simulink model "untitled1"  (Simulink 7.9)
settings: Solver=ode45  StartTime=0.0  StopTime=10.0  RelTol=1e-3
undefined symbols (not defined in the file or in its folder): b0, b1, b2, b3, Cyclic, D, dBW, F_nco, Fs, Hz, magnitude, N, nco_nominal, OFDM_Frame, sided, Ts, Two
libraries: dspobslib x17, dspsigops x8, simulink x8, dspsnks4 x4, dspxfrm3 x3, dspsrcs4 x3, dspstat3 x3, dspbuff3 x2, dsppolyfun x1, commrandsrc2 x1, commsink2 x1
settings Model: Creator=Estilo  LastModifiedBy=Estilo

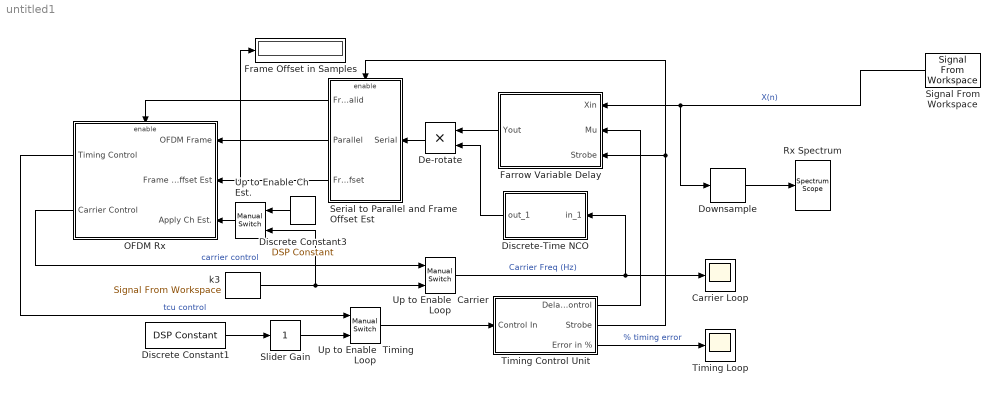
== system untitled1 ==
  Carrier Loop : Scope
      settings: TimeRange=0.008999999999999999  YMin=-1000  YMax=1000  MaxDataPoints=50000  Decimation=4
  De-rotate : Product  RndMeth=Zero
  Discrete Constant1 : dspobslib/DSP Constant  Value=nco_nominal  SampleMode=Discrete  discreteOutput=Sample-based (interpret vectors as 1-D)  continuousOutput=Sample-based  sampTime=2/F_nco  framePeriod=2/F_nco  dataType=Inherit via back propagation  isSigned=on  wordLen=16  udDataType=sfix(16)  fracBitsMode=Best precision  numFracBits=15  InterpretAs1D=on  Ts=2/F_nco  FramebasedOutput=off
      settings: additionalParams=on
  Discrete Constant3 : dspobslib/DSP Constant  Value=1  SampleMode=Discrete  discreteOutput=Sample-based (interpret vectors as 1-D)  continuousOutput=Sample-based  sampTime=inf  framePeriod=inf  dataType=Inherit via back propagation  isSigned=on  wordLen=16  udDataType=sfix(16)  fracBitsMode=Best precision  numFracBits=15  InterpretAs1D=on  Ts=inf  FramebasedOutput=off
      settings: additionalParams=on
  Discrete-Time NCO : Subsystem  mask(Discrete-Time VCO){Ac=1, Fc=0, Kc=1, Ph=0, ts=1/48000}
      mask prompts: Ac "Output amplitude:"; Fc "Oscillation frequency (Hz):"; Kc "Input sensitivity:"; Ph "Initial phase (rad):"; ts "Sample time:"
      mask help: Generate a discrete-time output signal whose frequency changes in response to the amplitude variations of the input signal. The input signal must be a scalar.
      mask init:
      | if ((length(Ac)~=1) | (length(Fc)~=1) | (length(Kc)~=1) | (length(Ph)~=1) | (length(ts)~=1) |(length(Ph)~=1))error('Mask parameters must be scalar values.');end;
      | pi2=2*pi;
      mask Help: helpview(commbhelp)
      mask Display: disp('Discrete-Time\nNCO (rab)')
  Downsample : dspsigops/Downsample  N=D/2  phase=0  InputProcessing=Inherited (this choice will be removed - see release notes)  RateOptions=Enforce single-rate processing  smode=Allow multirate  fmode=Maintain input frame size  ic=0
  Farrow Variable Delay : Subsystem
  Frame Offset in Samples : Display
  OFDM Rx : Subsystem
  Rx Spectrum : dspsnks4/Spectrum Scope  ScopeProperties=on  Domain=Frequency  HorizSpan=1  UseBuffer=on  BufferSize=80  Overlap=0  TreatMby1Signals=M channels  inpFftLenInherit=on  FFTlength=256  numAvg=10  DisplayProperties=off  AxisGrid=on  Memory=off  FrameNumber=on  AxisLegend=off  AxisZoom=off  OpenScopeAtSimStart=on  OpenScopeImmediately=off  FigPos=[623 549 194 174]  AxisProperties=off  XUnits=Hertz  XRange=Two-sided ((-Fs/2...Fs/2])  XDisplay=0  InheritXIncr=on  XIncr=1.0  XLabel=Samples  XLimit=Auto  YUnits=dBW/Hertz  XMax=1  XMin=0  YLabel=dBW/Hz  LineProperties=off  wintypeSpecScope=Boxcar  RsSpecScope=50  betaSpecScope=5  winsampSpecScope=Periodic  XAxisParamsVer=6.9  isFrameUpgraded=on
      settings: YMin=-79.4885  YMax=-44.4885
  Serial to Parallel and Frame Offset Est : Subsystem  TreatAsAtomicUnit=on
  Signal From Workspace : dspsrcs4/Signal From Workspace  X=yout1  Ts=1/48000  nsamps=320  OutputAfterFinalValue=Setting to zero  ignoreOrWarnInputAndFrameLengths=off
  Slider Gain : simulink/Math Operations/Slider Gain  low=0.99  gain=1  high=1.01
  Timing Control Unit : Subsystem
  Timing Loop : Scope
      settings: TimeRange=0.008999999999999999  YMin=-0.5  YMax=0.5  MaxDataPoints=50000
  Up to Enable  Carrier Loop : simulink/Signal Routing/Manual Switch  sw=0  action=0  varsize=off
  Up to Enable Ch Est. : simulink/Signal Routing/Manual Switch  sw=0  action=0  varsize=off
  Up to Enable  Timing Loop : simulink/Signal Routing/Manual Switch  sw=0  action=0  varsize=off
  k3 : dspsrcs4/Signal From Workspace  X=0  Ts=-1  nsamps=1  OutputAfterFinalValue=Holding final value  ignoreOrWarnInputAndFrameLengths=off
  wires:
  Timing Control Unit/1(Delay Control) -> Farrow Variable Delay/2(Mu)
  Timing Control Unit/2(Strobe) -> Farrow Variable Delay/3(Strobe), Serial to Parallel and Frame Offset Est/Enable
  Discrete Constant1/1 -> Slider Gain/1
  OFDM Rx/1(Timing Control) -> Up to Enable  Timing Loop/1  "tcu control"
  Up to Enable  Timing Loop/1 -> Timing Control Unit/1(Control In)
  Discrete-Time NCO/1(out_1) -> De-rotate/2
  De-rotate/1 -> Serial to Parallel and Frame Offset Est/1(Serial)
  Farrow Variable Delay/1(Yout) -> De-rotate/1
  Timing Control Unit/3(Error in %) -> Timing Loop/1  "% timing error"
  Downsample/1 -> Rx Spectrum/1
  Serial to Parallel and Frame Offset Est/2(Parallel) -> OFDM Rx/1(OFDM Frame)
  Serial to Parallel and Frame Offset Est/3(Frame Offset) -> OFDM Rx/2(Frame Offset Est), Frame Offset in Samples/1
  Slider Gain/1 -> Up to Enable  Timing Loop/2
  OFDM Rx/2(Carrier Control) -> Up to Enable  Carrier Loop/1  "carrier control"
  Up to Enable  Carrier Loop/1 -> Discrete-Time NCO/1(in_1), Carrier Loop/1  "Carrier Freq (Hz)"
  k3/1 -> Up to Enable  Carrier Loop/2, Up to Enable Ch Est./2
  Serial to Parallel and Frame Offset Est/1(FrameValid) -> OFDM Rx/Enable
  Up to Enable Ch Est./1 -> OFDM Rx/3(Apply Ch Est.)
  Discrete Constant3/1 -> Up to Enable Ch Est./1
  Signal From Workspace/1 -> Farrow Variable Delay/1(Xin), Downsample/1  "X(n)"

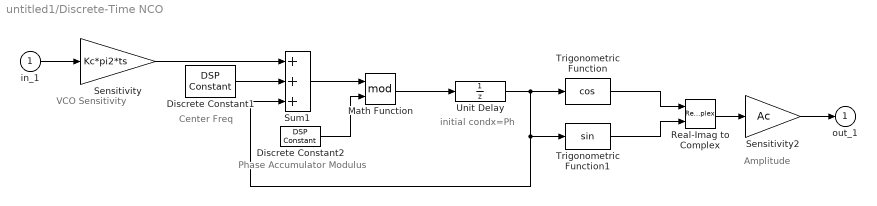
== system untitled1/Discrete-Time NCO ==
  note: Amplitude
  note: Phase Accumulator
      | Modulus
  note: Center Freq
  note: VCO Sensitivity
  note: initial condx=Ph
  in_1 : Inport
  Discrete Constant1 : dspobslib/DSP Constant  Value=Fc*pi2*ts  SampleMode=Discrete  discreteOutput=Sample-based (interpret vectors as 1-D)  continuousOutput=Sample-based  sampTime=ts  framePeriod=ts  dataType=Inherit via back propagation  isSigned=on  wordLen=16  udDataType=sfix(16)  fracBitsMode=Best precision  numFracBits=15  InterpretAs1D=on  Ts=ts  FramebasedOutput=off
      settings: additionalParams=on
  Discrete Constant2 : dspobslib/DSP Constant  Value=pi2  SampleMode=Discrete  discreteOutput=Sample-based (interpret vectors as 1-D)  continuousOutput=Sample-based  sampTime=ts  framePeriod=ts  dataType=Inherit via back propagation  isSigned=on  wordLen=16  udDataType=sfix(16)  fracBitsMode=Best precision  numFracBits=15  InterpretAs1D=on  Ts=ts  FramebasedOutput=off
      settings: additionalParams=on
  Math Function : Math  Operator=mod  SaturateOnIntegerOverflow=on
  Real-Imag to Complex : RealImagToComplex
  Sensitivity : Gain  Gain=Kc*pi2*ts  SaturateOnIntegerOverflow=on  OutDataTypeStr=Inherit: Same as input  ParamDataTypeStr=Inherit: Same as input
  Sensitivity2 : Gain  Gain=Ac  SaturateOnIntegerOverflow=on  OutDataTypeStr=Inherit: Same as input  ParamDataTypeStr=Inherit: Same as input
  Sum1 : Sum  Inputs=+++  SaturateOnIntegerOverflow=on  InputSameDT=on  OutDataTypeStr=Inherit: Same as first input
  Trigonometric Function : Trigonometry  Operator=cos
  Trigonometric Function1 : Trigonometry
  Unit Delay : UnitDelay  X0=Ph  SampleTime=ts
  out_1 : Outport  InitialOutput=0
  wires:
  Discrete Constant1/1 -> Sum1/2
  Sensitivity2/1 -> out_1/1
  Trigonometric Function/1 -> Real-Imag to Complex/1
  Unit Delay/1 -> Sum1/3, Trigonometric Function1/1, Trigonometric Function/1
  Sensitivity/1 -> Sum1/1
  in_1/1 -> Sensitivity/1
  Math Function/1 -> Unit Delay/1
  Sum1/1 -> Math Function/1
  Discrete Constant2/1 -> Math Function/2
  Trigonometric Function1/1 -> Real-Imag to Complex/2
  Real-Imag to Complex/1 -> Sensitivity2/1

== system untitled1/Farrow Variable Delay ==
  Xin : Inport
  Mu : Inport  Port=2
  Strobe : Inport  Port=3
  Calculate Filter : Subsystem
  Filter State (4x1) : Buffer  N=4  V=3
  Yout : Outport
  wires:
  Xin/1 -> Filter State (4x1)/1
  Mu/1 -> Calculate Filter/1(In1)
  Filter State (4x1)/1 -> Calculate Filter/2(In2)
  Calculate Filter/1(Out1) -> Yout/1
  Strobe/1 -> Calculate Filter/Enable

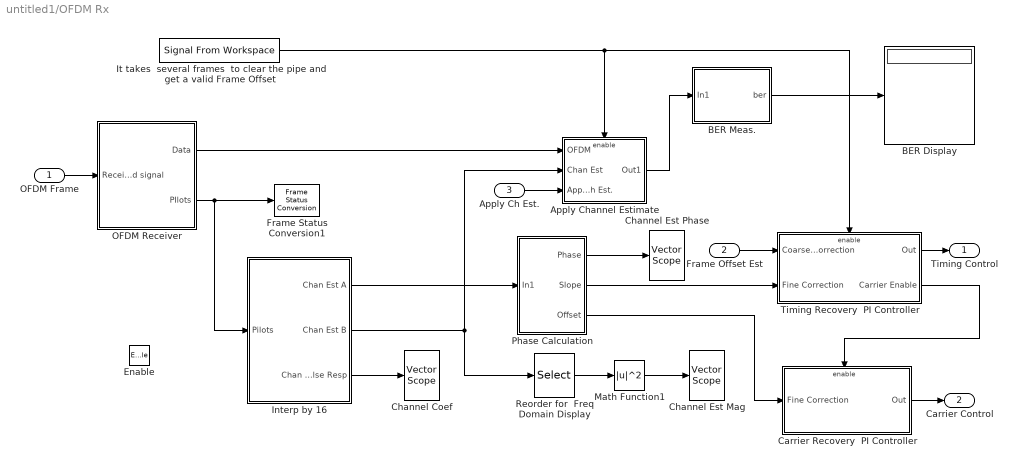
== system untitled1/OFDM Rx ==
  OFDM Frame : Inport
  Frame Offset Est : Inport  Port=2
  Apply Ch Est. : Inport  Port=3
  Enable : EnablePort
  Apply Channel Estimate : Subsystem
  BER Display : Display
  BER Meas. : Subsystem
  Carrier Recovery  PI Controller : Subsystem
  Channel Coef : dspsnks4/Vector Scope  ScopeProperties=on  Domain=Time  HorizSpan=1  DisplayProperties=off  AxisGrid=on  Memory=off  FrameNumber=off  AxisLegend=off  AxisZoom=off  OpenScopeAtSimStart=on  OpenScopeImmediately=off  FigPos=[827 549 193 173]  AxisProperties=off  XUnits=Hertz  XRange=[0...Fs/2]  InheritXIncr=on  XIncr=1  XLabel=Time  XLimit=Auto  XMin=0  XMax=1  XStart=0  YUnits=dB  YLabel=Amplitude  LineProperties=off  LineStyles=none|none  LineMarkers=*|*  LineColors=blue | red  XAxisParamsVer=6.9
      settings: YMin=-2  YMax=2
  "Channel Est Mag " : dspsnks4/Vector Scope  ScopeProperties=on  Domain=Frequency  HorizSpan=1  DisplayProperties=off  AxisGrid=on  Memory=off  FrameNumber=on  AxisLegend=off  AxisZoom=off  OpenScopeAtSimStart=on  OpenScopeImmediately=off  FigPos=[624 329 193 172]  AxisProperties=off  XUnits=Hertz  XRange=[-Fs/2...Fs/2]  InheritXIncr=off  XIncr=8/F_nco  XLabel=Time  XLimit=Auto  XMin=0  XMax=1  XStart=0  YUnits=dB  YLabel=Amplitude in dB  LineProperties=off  XAxisParamsVer=6.9
      settings: YMin=-20  YMax=15
  Channel Est Phase : dspsnks4/Vector Scope  ScopeProperties=on  Domain=Frequency  HorizSpan=1  DisplayProperties=off  AxisGrid=on  Memory=off  FrameNumber=off  AxisLegend=off  AxisZoom=off  OpenScopeAtSimStart=on  OpenScopeImmediately=off  FigPos=[827 332 196 169]  AxisProperties=off  XUnits=Hertz  XRange=[-Fs/2...Fs/2]  InheritXIncr=off  XIncr=8/F_nco  XLabel=Time  XLimit=Auto  XMin=0  XMax=1  XStart=0  YUnits=Magnitude  YLabel=Degrees  LineProperties=off  LineColors=blue  XAxisParamsVer=6.9
      settings: YMin=-400  YMax=400
  Frame Status Conversion1 : dspobslib/Frame Status Conversion  growRefPort=off  outframe=Frame-based
  Interp by 16 : Subsystem
  It takes  several frames  to clear the pipe and get a valid Frame Offset : dspsrcs4/Signal From Workspace  X=[zeros(1,10),1]  Ts=-1  nsamps=1  OutputAfterFinalValue=Holding final value  ignoreOrWarnInputAndFrameLengths=off
  Math Function1 : Math  Operator=magnitude^2  SaturateOnIntegerOverflow=on
  OFDM Receiver : Subsystem
      mask Display:
      | disp('OFDM\nReceiver');
      | port_label('output',2,'pilots')
  Phase Calculation : Subsystem
  Reorder for  Freq Domain Display : Selector  InputPortWidth=128  IndexOptions=Index vector (dialog)  Indices=[65:128 1:64]  OutputSizes=1
  Timing Recovery  PI Controller : Subsystem
  Timing Control : Outport  InitialOutput=nco_nominal
  Carrier Control : Outport  Port=2  InitialOutput=0
  wires:
  OFDM Frame/1 -> OFDM Receiver/1(Received signal)
  OFDM Receiver/2(PIlots) -> Interp by 16/1(Pilots), Frame Status Conversion1/1
  Interp by 16/2(Chan Est B) -> Apply Channel Estimate/2(Chan Est), Reorder for  Freq Domain Display/1
  Reorder for  Freq Domain Display/1 -> Math Function1/1
  Phase Calculation/2(Slope) -> Timing Recovery  PI Controller/2(Fine Correction)
  OFDM Receiver/1(Data) -> Apply Channel Estimate/1(OFDM)
  Phase Calculation/1(Phase) -> Channel Est Phase/1
  Math Function1/1 -> "Channel Est Mag "/1
  Timing Recovery  PI Controller/1(Out) -> Timing Control/1
  It takes  several frames  to clear the pipe and get a valid Frame Offset/1 -> Apply Channel Estimate/Enable, Timing Recovery  PI Controller/Enable
  Carrier Recovery  PI Controller/1(Out) -> Carrier Control/1
  Frame Offset Est/1 -> Timing Recovery  PI Controller/1(Coarse Correction)
  Phase Calculation/3(Offset) -> Carrier Recovery  PI Controller/1(Fine Correction)
  Interp by 16/3(Chan Impulse Resp) -> Channel Coef/1
  Interp by 16/1(Chan Est A) -> Phase Calculation/1(In1)
  Apply Channel Estimate/1(Out1) -> BER Meas./1(In1)
  Apply Ch Est./1 -> Apply Channel Estimate/3(Apply Ch Est.)
  Timing Recovery  PI Controller/2(Carrier Enable) -> Carrier Recovery  PI Controller/Enable
  BER Meas./1(ber) -> BER Display/1

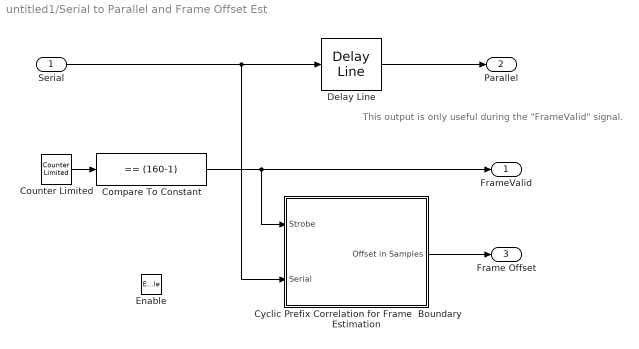
== system untitled1/Serial to Parallel and Frame Offset Est ==
  note: This output is only
      | useful during the "FrameValid" signal.
  Serial : Inport
  Enable : EnablePort
  Compare To Constant : simulink/Logic and Bit Operations/Compare To Constant  relop===  const=(160-1)  OutDataTypeStr=boolean  ZeroCross=off
  Counter Limited : simulink/Sources/Counter Limited  uplimit=(160-1)  tsamp=-1
  Cyclic Prefix Correlation for Frame  Boundary Estimation : Subsystem
  Delay Line : dspbuff3/Delay Line  siz=160  ic=0  directfeed=on  enable_output=off  hold_output=off  TreatMby1Signals=M channels (this choice will be removed - see release notes)
  FrameValid : Outport  OutputWhenDisabled=reset  InitialOutput=0
  Parallel : Outport  Port=2
  Frame Offset : Outport  Port=3
  wires:
  Serial/1 -> Delay Line/1, Cyclic Prefix Correlation for Frame  Boundary Estimation/2(Serial)
  Counter Limited/1 -> Compare To Constant/1
  Delay Line/1 -> Parallel/1
  Compare To Constant/1 -> FrameValid/1, Cyclic Prefix Correlation for Frame  Boundary Estimation/1(Strobe)
  Cyclic Prefix Correlation for Frame  Boundary Estimation/1(Offset in Samples) -> Frame Offset/1

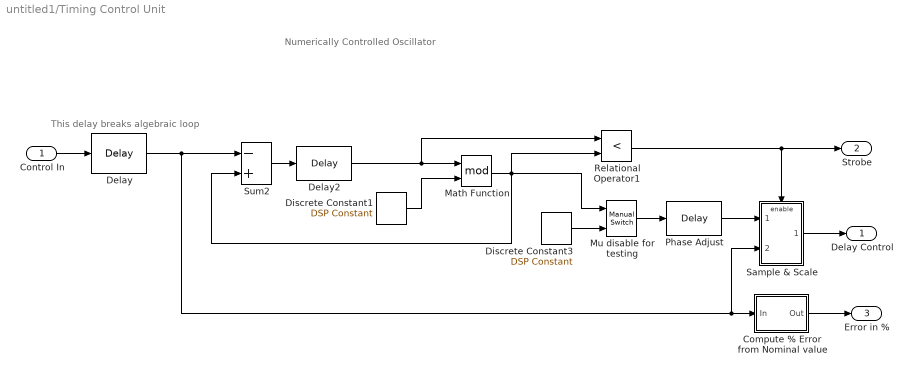
== system untitled1/Timing Control Unit ==
  note: Numerically Controlled Oscillator
  note: This delay breaks algebraic loop
  Control In : Inport
  Compute % Error from Nominal value : Subsystem
  Delay : dspsigops/Delay  InputProcessing=Inherited (this choice will be removed - see release notes)  dly_unit=Samples  delay=1  ic_detail=off  dif_ic_for_ch=off  dif_ic_for_dly=off  ic=nco_nominal  reset_popup=None
  Delay2 : dspsigops/Delay  InputProcessing=Inherited (this choice will be removed - see release notes)  dly_unit=Samples  delay=1  ic_detail=on  dif_ic_for_ch=off  dif_ic_for_dly=off  ic=0  reset_popup=None
  Discrete Constant1 : dspobslib/DSP Constant  Value=1  SampleMode=Discrete  discreteOutput=Sample-based (interpret vectors as 1-D)  continuousOutput=Sample-based  sampTime=inf  framePeriod=inf  dataType=Inherit via back propagation  isSigned=on  wordLen=16  udDataType=sfix(16)  fracBitsMode=Best precision  numFracBits=15  InterpretAs1D=on  Ts=inf  FramebasedOutput=off
      settings: additionalParams=on
  Discrete Constant3 : dspobslib/DSP Constant  Value=0  SampleMode=Discrete  discreteOutput=Sample-based (interpret vectors as 1-D)  continuousOutput=Sample-based  sampTime=inf  framePeriod=inf  dataType=Inherit via back propagation  isSigned=on  wordLen=16  udDataType=sfix(16)  fracBitsMode=Best precision  numFracBits=15  InterpretAs1D=on  Ts=inf  FramebasedOutput=off
      settings: additionalParams=on
  Math Function : Math  Operator=mod  SaturateOnIntegerOverflow=on
  Mu disable for testing : simulink/Signal Routing/Manual Switch  sw=1  action=0  varsize=off
  Phase Adjust : dspsigops/Delay  InputProcessing=Inherited (this choice will be removed - see release notes)  dly_unit=Samples  delay=1  ic_detail=on  dif_ic_for_ch=off  dif_ic_for_dly=off  ic=0  reset_popup=None
  Relational Operator1 : RelationalOperator  Operator=<  OutDataTypeStr=boolean
  Sample & Scale : Subsystem
  Sum2 : Sum  Inputs=-+  SaturateOnIntegerOverflow=on  InputSameDT=on  OutDataTypeStr=Inherit: Same as first input
  Delay Control : Outport
  Strobe : Outport  Port=2
  Error in % : Outport  Port=3
  wires:
  Relational Operator1/1 -> Sample & Scale/Enable, Strobe/1
  Math Function/1 -> Relational Operator1/2, Sum2/2, Mu disable for testing/1
  Sum2/1 -> Delay2/1
  Discrete Constant1/1 -> Math Function/2
  Delay2/1 -> Relational Operator1/1, Math Function/1
  Control In/1 -> Delay/1
  Mu disable for testing/1 -> Phase Adjust/1
  Sample & Scale/1(Out1) -> Delay Control/1
  Phase Adjust/1 -> Sample & Scale/1(In1)
  Discrete Constant3/1 -> Mu disable for testing/2
  Delay/1 -> Sum2/1, Sample & Scale/2(In2), Compute % Error from Nominal value/1(In)
  Compute % Error from Nominal value/1(Out) -> Error in %/1

== system untitled1/Farrow Variable Delay/Calculate Filter ==
  note: Filter Coefficients from Chris Dick Xilinx,
      | or H. Meyer pp 520 (9-33) Digital Communications Receivers
  In1 : Inport
  In2 : Inport  Port=2
  Enable : EnablePort
  Filter coefficients : Gain  Gain=fliplr([b3;b2;b1;b0])  Multiplication=Matrix(K*u)  SaturateOnIntegerOverflow=on  OutDataTypeStr=Inherit: Same as input  ParamDataTypeStr=Inherit: Same as input
  Polynomial Evaluation : dsppolyfun/Polynomial Evaluation  useConstCoeffs=off  constCoeffs=[5 4 3 2 1]
  Out1 : Outport
  wires:
  In1/1 -> Polynomial Evaluation/1
  Polynomial Evaluation/1 -> Out1/1
  In2/1 -> Filter coefficients/1
  Filter coefficients/1 -> Polynomial Evaluation/2

== system untitled1/OFDM Rx/Apply Channel Estimate ==
  note: Extract Matching Channel
      | Corrections
  OFDM : Inport
  Chan Est : Inport  Port=2
  Apply Ch Est. : Inport  Port=3
  Enable : EnablePort
  Divide : Product  Inputs=*/  RndMeth=Zero
  Frame Status Conversion2 : dspobslib/Frame Status Conversion  growRefPort=off  outframe=Frame-based
  Selector : Selector  InputPortWidth=128  IndexOptions=Index vector (dialog)  Indices=[57 59 61 63 67 69 71 73 ]  OutputSizes=1
  Switch : Switch  Threshold=.5
  Out1 : Outport
  wires:
  Selector/1 -> Divide/2
  OFDM/1 -> Divide/1, Switch/3
  Chan Est/1 -> Selector/1
  Switch/1 -> Frame Status Conversion2/1
  Divide/1 -> Switch/1
  Apply Ch Est./1 -> Switch/2
  Frame Status Conversion2/1 -> Out1/1

== system untitled1/OFDM Rx/BER Meas. ==
  In1 : Inport
  Bernoulli Random Binary Generator : commrandsrc2/Bernoulli Binary Generator  P=0.5  seed=123  Ts=1/1000  frameBased=on  sampPerFrame=4  orient=off  outDataType=double
  Error Rate Calculation : commsink2/Error Rate Calculation  N=270  st_delay=810-180  cp_mode=Entire frame  subframe=[]  PMode=Port  WsName=ErrorVec  RsMode2=off  stop=off  numErr=100  maxBits=1e6
  ber : Outport  InitialOutput=nco_nominal
  wires:
  Bernoulli Random Binary Generator/1 -> Error Rate Calculation/1
  In1/1 -> Error Rate Calculation/2
  Error Rate Calculation/1 -> ber/1

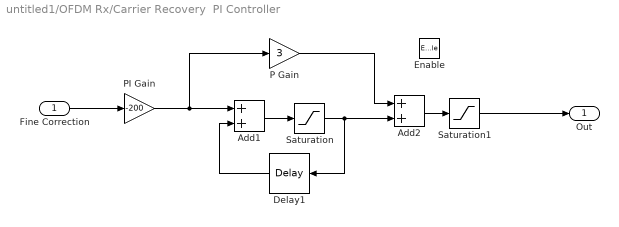
== system untitled1/OFDM Rx/Carrier Recovery  PI Controller ==
  Fine Correction : Inport
  Enable : EnablePort
  Add1 : Sum
  Add2 : Sum
  Delay1 : dspsigops/Delay  InputProcessing=Inherited (this choice will be removed - see release notes)  dly_unit=Samples  delay=1  ic_detail=off  dif_ic_for_ch=off  dif_ic_for_dly=off  ic=0  reset_popup=None
  P Gain : Gain  Gain=3
  PI Gain : Gain  Gain=-200
  Saturation : Saturate  UpperLimit=2000  LowerLimit=-2000
  Saturation1 : Saturate  UpperLimit=2000  LowerLimit=-2000
  Out : Outport
  wires:
  P Gain/1 -> Add2/1
  Add2/1 -> Saturation1/1
  Fine Correction/1 -> PI Gain/1
  PI Gain/1 -> P Gain/1, Add1/1
  Saturation/1 -> Add2/2, Delay1/1
  Add1/1 -> Saturation/1
  Delay1/1 -> Add1/2
  Saturation1/1 -> Out/1

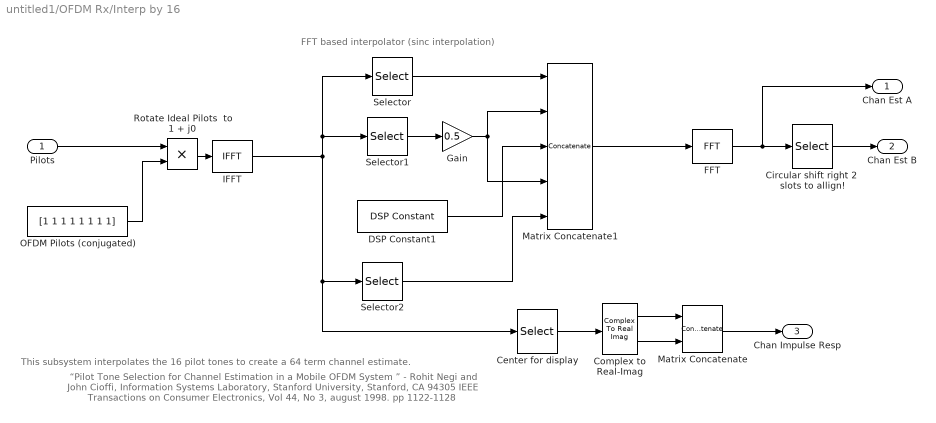
== system untitled1/OFDM Rx/Interp by 16 ==
  note: FFT based interpolator (sinc interpolation)
  note: This subsystem interpolates the 16 pilot
      |  tones to create a 64 term channel estimate.
  note: “Pilot Tone Selection for Channel Estimation in a Mobile OFDM System ”
      | -  Rohit Negi and John Cioffi, Information Systems Laboratory, Stanford University, Stanford, CA 94305
      | IEEE Transactions on Consumer Electronics, Vol 44, No 3, august 1998. pp 1122-1128
  Pilots : Inport
  "Center for display " : Selector  InputPortWidth=8  IndexOptions=Index vector (dialog)  Indices=[5:8 1:4]  OutputSizes=1
  Circular shift right 2  slots to allign! : Selector  InputPortWidth=128  IndexOptions=Index vector (dialog)  Indices=[127 128 1:126]  OutputSizes=1
  Complex to Real-Imag : ComplexToRealImag
  DSP Constant1 : dspobslib/DSP Constant  Value=zeros(119,1)  SampleMode=Discrete  discreteOutput=Sample-based  continuousOutput=Sample-based  sampTime=-1  framePeriod=2  dataType=Inherit from 'Constant value'  isSigned=on  wordLen=16  udDataType=sfix(16)  fracBitsMode=Best precision  numFracBits=15  InterpretAs1D=-inf  Ts=-inf  FramebasedOutput=-inf
  FFT : dspxfrm3/FFT  CompMethod=Table lookup  TableOpt=HYBRID  TableOptActive=Speed  BitRevOrder=off  InheritFFTLength=on  FFTLength=64  RowConvenienceOn=on  FFTImplementation=Auto  SkipNorm=off  firstCoeffDataTypeStr=Inherit: Same word length as input  firstCoeffLastDataTypeStr=Inherit: Same word length as input  outputMin=[]  outputMax=[]  roundingMode=Floor  overflowMode=off
  Gain : Gain  Gain=0.5
  IFFT : dspxfrm3/IFFT  CompMethod=Table lookup  TableOpt=HYBRID  TableOptActive=Speed  BitRevOrder=off  cs_in=off  SkipNorm=on  InheritFFTLength=on  FFTLength=64  mode=Complex  outSamplingMode=Frame based  RowConvenienceOn=on  FFTImplementation=Auto  firstCoeffDataTypeStr=Inherit: Same word length as input  firstCoeffLastDataTypeStr=Inherit: Same word length as input  outputMin=[]  outputMax=[]  roundingMode=Floor  overflowMode=off
  Matrix Concatenate : Concatenate  Mode=Multidimensional array  ConcatenateDimension=2
  Matrix Concatenate1 : Concatenate  NumInputs=5  Mode=Multidimensional array
  OFDM Pilots (conjugated) : Constant  Value=[1 1 1 1 1 1 1 1]  FramePeriod=-1
  Rotate Ideal Pilots  to 1 + j0 : Product  Inputs=**  RndMeth=Zero
  Selector : Selector  InputPortWidth=8  IndexOptions=Index vector (dialog)  Indices=[1:4]  OutputSizes=1
  Selector1 : Selector  InputPortWidth=8  IndexOptions=Index vector (dialog)  Indices=5  OutputSizes=1
  Selector2 : Selector  InputPortWidth=8  IndexOptions=Index vector (dialog)  Indices=6:8  OutputSizes=1
  Chan Est A : Outport
  Chan Est B : Outport  Port=2
  Chan Impulse Resp : Outport  Port=3
  wires:
  Matrix Concatenate1/1 -> FFT/1
  Selector/1 -> Matrix Concatenate1/1
  Selector1/1 -> Gain/1
  DSP Constant1/1 -> Matrix Concatenate1/3
  Gain/1 -> Matrix Concatenate1/2, Matrix Concatenate1/4
  Selector2/1 -> Matrix Concatenate1/5
  FFT/1 -> Chan Est A/1, Circular shift right 2  slots to allign!/1
  IFFT/1 -> Selector/1, Selector1/1, Selector2/1, "Center for display "/1
  Complex to Real-Imag/1 -> Matrix Concatenate/1
  Complex to Real-Imag/2 -> Matrix Concatenate/2
  "Center for display "/1 -> Complex to Real-Imag/1
  Matrix Concatenate/1 -> Chan Impulse Resp/1
  Circular shift right 2  slots to allign!/1 -> Chan Est B/1
  Rotate Ideal Pilots  to 1 + j0/1 -> IFFT/1
  Pilots/1 -> Rotate Ideal Pilots  to 1 + j0/1
  OFDM Pilots (conjugated)/1 -> Rotate Ideal Pilots  to 1 + j0/2

== system untitled1/OFDM Rx/OFDM Receiver ==
  Received signal : Inport
  FFT : dspxfrm3/FFT  CompMethod=Table lookup  TableOpt=HYBRID  TableOptActive=Speed  BitRevOrder=off  InheritFFTLength=on  FFTLength=64  RowConvenienceOn=on  FFTImplementation=Auto  SkipNorm=off  firstCoeffDataTypeStr=Inherit: Same word length as input  firstCoeffLastDataTypeStr=Inherit: Same word length as input  outputMin=[]  outputMax=[]  roundingMode=Floor  overflowMode=off
  Gain1 : Gain  Gain=1/8
  Gain2 : Gain  Gain=1/6  SaturateOnIntegerOverflow=on  OutDataTypeStr=Inherit: Same as input  ParamDataTypeStr=Inherit: Same as input
  Remove Cyclic Prefix : Selector  InputPortWidth=160  IndexOptions=Index vector (dialog)  Indices=[33:160]  OutputSizes=1
  Remove pilots : Subsystem
  reorder : Selector  InputPortWidth=128  IndexOptions=Index vector (dialog)  Indices=[65:128 1:64]  OutputSizes=1
  Data : Outport
  PIlots : Outport  Port=2
  wires:
  FFT/1 -> reorder/1
  Received signal/1 -> Remove Cyclic Prefix/1
  Remove Cyclic Prefix/1 -> FFT/1
  Remove pilots/2(Pilots) -> Gain1/1
  Remove pilots/1(Data) -> Gain2/1
  Gain2/1 -> Data/1
  reorder/1 -> Remove pilots/1("  ")
  Gain1/1 -> PIlots/1

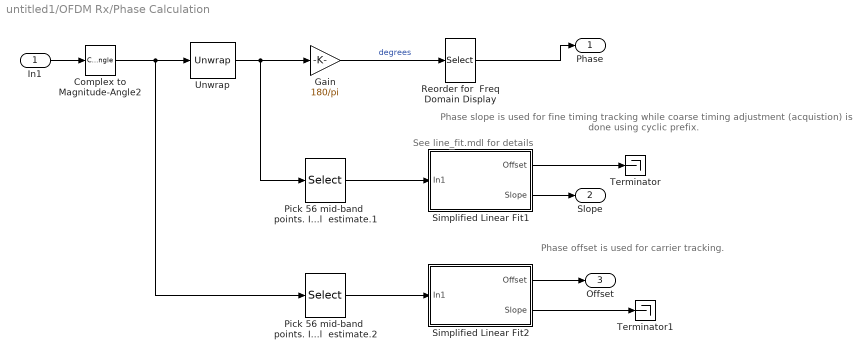
== system untitled1/OFDM Rx/Phase Calculation ==
  note: See line_fit.mdl for details
  note: Phase slope is used for fine
      | timing tracking while coarse timing adjustment
      | (acquistion) is done using cyclic prefix.
  note: Phase offset is used for carrier tracking.
  In1 : Inport
  Complex to Magnitude-Angle2 : ComplexToMagnitudeAngle  Output=Angle
  Gain : Gain  Gain=180/pi
  Pick 56 mid-band  points. Ignore end points of channel  estimate.1 : Selector  InputPortWidth=128  IndexOptions=Index vector (dialog)  Indices=[37:92]  OutputSizes=1
  Pick 56 mid-band  points. Ignore end points of channel  estimate.2 : Selector  InputPortWidth=128  IndexOptions=Index vector (dialog)  Indices=[[37:92]]  OutputSizes=1
  Reorder for  Freq Domain Display : Selector  InputPortWidth=128  IndexOptions=Index vector (dialog)  Indices=[65:128 1:64]  OutputSizes=1
  Simplified Linear Fit1 : Subsystem
  Simplified Linear Fit2 : Subsystem
  Terminator : Terminator
  Terminator1 : Terminator
  Unwrap : dspsigops/Unwrap  tol=pi*1.99 %1.9  InputProcessing=Inherited (this choice will be removed - see release notes)  running=on
  Phase : Outport
  Slope : Outport  Port=2
  Offset : Outport  Port=3
  wires:
  Complex to Magnitude-Angle2/1 -> Unwrap/1, Pick 56 mid-band  points. Ignore end points of channel  estimate.2/1
  In1/1 -> Complex to Magnitude-Angle2/1
  Gain/1 -> Reorder for  Freq Domain Display/1  "degrees"
  Reorder for  Freq Domain Display/1 -> Phase/1
  Pick 56 mid-band  points. Ignore end points of channel  estimate.1/1 -> Simplified Linear Fit1/1(In1)
  Simplified Linear Fit1/2(Slope) -> Slope/1
  Unwrap/1 -> Gain/1, Pick 56 mid-band  points. Ignore end points of channel  estimate.1/1
  Pick 56 mid-band  points. Ignore end points of channel  estimate.2/1 -> Simplified Linear Fit2/1(In1)
  Simplified Linear Fit2/1(Offset) -> Offset/1
  Simplified Linear Fit1/1(Offset) -> Terminator/1
  Simplified Linear Fit2/2(Slope) -> Terminator1/1

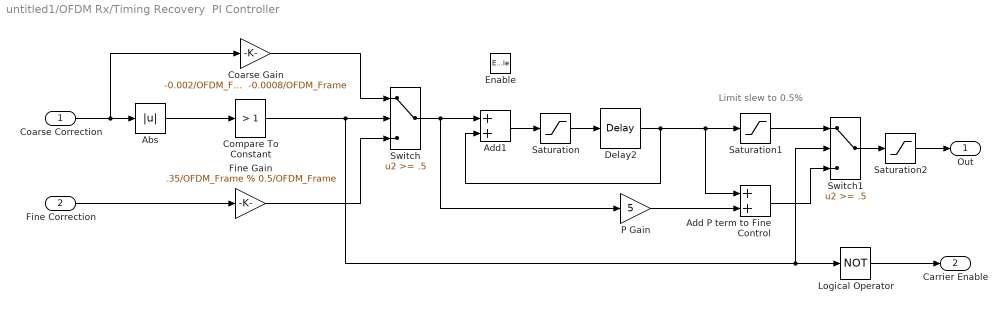
== system untitled1/OFDM Rx/Timing Recovery  PI Controller ==
  note: Limit slew to 0.5%
  Coarse Correction : Inport
  Fine Correction : Inport  Port=2
  Enable : EnablePort
  Abs : Abs
  Add P term to Fine Control : Sum
  Add1 : Sum
  Coarse Gain : Gain  Gain="-0.002/OFDM_Frame   %  -0.0008/OFDM_Frame"
  Compare To Constant : simulink/Logic and Bit Operations/Compare To Constant  relop=>  const=1  OutDataTypeStr=boolean  ZeroCross=off
  Delay2 : dspsigops/Delay  InputProcessing=Inherited (this choice will be removed - see release notes)  dly_unit=Samples  delay=1  ic_detail=off  dif_ic_for_ch=off  dif_ic_for_dly=off  ic=nco_nominal  reset_popup=None
  Fine Gain : Gain  Gain=.35/OFDM_Frame % 0.5/OFDM_Frame
  Logical Operator : Logic  Operator=NOT  AllPortsSameDT=off  OutDataTypeStr=boolean
  P Gain : Gain  Gain=5
  Saturation : Saturate  UpperLimit=nco_nominal*1.005  LowerLimit=nco_nominal*0.995
  Saturation1 : Saturate  UpperLimit=nco_nominal*1.005  LowerLimit=nco_nominal*0.995
  Saturation2 : Saturate  UpperLimit="nco_nominal*1.007  % 1.007"  LowerLimit="nco_nominal*0.993  % 0.993"
  Switch : Switch  Threshold=.5
  Switch1 : Switch  Threshold=.5
  Out : Outport
  Carrier Enable : Outport  Port=2
  wires:
  Add1/1 -> Saturation/1
  Switch/1 -> Add1/1, P Gain/1
  Coarse Gain/1 -> Switch/1
  Fine Gain/1 -> Switch/3
  Coarse Correction/1 -> Abs/1, Coarse Gain/1
  Fine Correction/1 -> Fine Gain/1
  Abs/1 -> Compare To Constant/1
  Delay2/1 -> Add1/2, Add P term to Fine Control/1, Saturation1/1
  P Gain/1 -> Add P term to Fine Control/2
  Add P term to Fine Control/1 -> Switch1/3
  Switch1/1 -> Saturation2/1
  Compare To Constant/1 -> Switch/2, Switch1/2, Logical Operator/1
  Saturation2/1 -> Out/1
  Logical Operator/1 -> Carrier Enable/1
  Saturation/1 -> Delay2/1
  Saturation1/1 -> Switch1/1

== system untitled1/Serial to Parallel and Frame Offset Est/Cyclic Prefix Correlation for Frame  Boundary Estimation ==
  note: http://citeseer.ist.psu.edu/cache/papers/cs/27222/http:zSzzSzwww.sm.luth.sezSzcseezSzspzSzresearchzSzconferencezSzbsb96c.pdf/on-synchronization-in-ofdm.pdf
  note: Google " On Synchronization in OFDM Systems Using the Cyclic Prefix "
  Strobe : Inport
  Serial : Inport  Port=2
  Estimators : Subsystem
  Find max : Subsystem
  Terminator : Terminator
  buffer one frame worth : dspbuff3/Delay Line  siz=160  ic=0  directfeed=on  enable_output=off  hold_output=off  TreatMby1Signals=M channels (this choice will be removed - see release notes)
  Offset in Samples : Outport
  wires:
  Estimators/1(Delay Est Data) -> buffer one frame worth/1
  buffer one frame worth/1 -> Find max/1(In1)
  Estimators/2(Freq Error Est) -> Terminator/1
  Strobe/1 -> Find max/Enable
  Serial/1 -> Estimators/1(In1)
  Find max/1(Frame Offset Est) -> Offset in Samples/1

== system untitled1/Timing Control Unit/Compute % Error from Nominal value ==
  In : Inport
  Add : Sum  Inputs=+-
  Discrete Constant3 : dspobslib/DSP Constant  Value=1  SampleMode=Discrete  discreteOutput=Sample-based (interpret vectors as 1-D)  continuousOutput=Sample-based  sampTime=2/F_nco  framePeriod=2/F_nco  dataType=Inherit via back propagation  isSigned=on  wordLen=16  udDataType=sfix(16)  fracBitsMode=Best precision  numFracBits=15  InterpretAs1D=on  Ts=2/F_nco  FramebasedOutput=off
      settings: additionalParams=on
  Gain : Gain  Gain=1/nco_nominal
  Gain1 : Gain  Gain=100
  Out : Outport
  wires:
  Gain1/1 -> Out/1
  In/1 -> Gain/1
  Discrete Constant3/1 -> Add/2
  Add/1 -> Gain1/1
  Gain/1 -> Add/1

== system untitled1/Timing Control Unit/Sample & Scale ==
  In1 : Inport
  In2 : Inport  Port=2
  Enable : EnablePort
  Discrete Constant2 : dspobslib/DSP Constant  Value=-1  SampleMode=Discrete  discreteOutput=Sample-based (interpret vectors as 1-D)  continuousOutput=Sample-based  sampTime=inf  framePeriod=inf  dataType=Inherit via back propagation  isSigned=on  wordLen=16  udDataType=sfix(16)  fracBitsMode=Best precision  numFracBits=15  InterpretAs1D=on  Ts=inf  FramebasedOutput=off
      settings: additionalParams=on
  Product : Product  Inputs=*/  RndMeth=Zero
  Sum1 : Sum  SaturateOnIntegerOverflow=on  InputSameDT=on  OutDataTypeStr=Inherit: Same as first input
  Out1 : Outport
  wires:
  Product/1 -> Sum1/1
  Discrete Constant2/1 -> Sum1/2
  In1/1 -> Product/1
  Sum1/1 -> Out1/1
  In2/1 -> Product/2

== system untitled1/OFDM Rx/OFDM Receiver/Remove pilots ==
  note: Get Data Sans
      | 3 Zero Channels
  "  " : Inport
  Selector : Selector  InputPortWidth=128  IndexOptions=Index vector (dialog)  Indices="[  58 60 62 64 66 68 70 72 ]"  OutputSizes=1
  Selector1 : Selector  InputPortWidth=128  IndexOptions=Index vector (dialog)  Indices=[57 59 61 63 67 69 71 73 ]  OutputSizes=1
  Data : Outport
  Pilots : Outport  Port=2
  wires:
  "  "/1 -> Selector/1, Selector1/1
  Selector/1 -> Data/1
  Selector1/1 -> Pilots/1

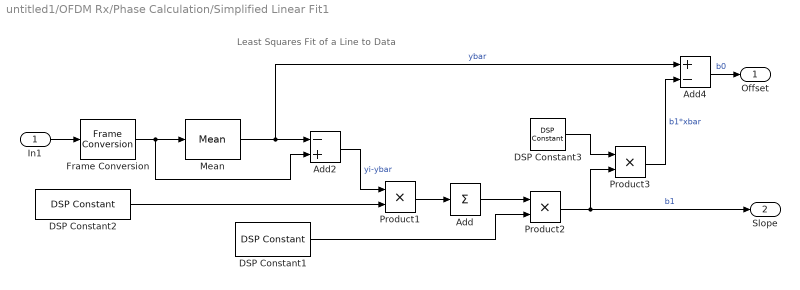
== system untitled1/OFDM Rx/Phase Calculation/Simplified Linear Fit1 ==
  note: Least Squares Fit of a Line to Data
  In1 : Inport
  Add : Sum  Inputs=+
  Add2 : Sum  Inputs=-+
  Add4 : Sum  Inputs=+-
  DSP Constant1 : dspobslib/DSP Constant  Value=1/14630  SampleMode=Discrete  discreteOutput=Sample-based  continuousOutput=Sample-based  sampTime=inf  framePeriod=N*Ts  dataType=Inherit from 'Constant value'  isSigned=on  wordLen=16  udDataType=sfix(16)  fracBitsMode=Best precision  numFracBits=15  InterpretAs1D=-inf  Ts=-inf  FramebasedOutput=-inf
  DSP Constant2 : dspobslib/DSP Constant  Value=[-27.5:27.5]'  SampleMode=Discrete  discreteOutput=Sample-based  continuousOutput=Sample-based  sampTime=inf  framePeriod=N*Ts  dataType=Inherit from 'Constant value'  isSigned=on  wordLen=16  udDataType=sfix(16)  fracBitsMode=Best precision  numFracBits=15  InterpretAs1D=-inf  Ts=-inf  FramebasedOutput=-inf
  DSP Constant3 : dspobslib/DSP Constant  Value=-.5  SampleMode=Discrete  discreteOutput=Sample-based  continuousOutput=Sample-based  sampTime=inf  framePeriod=N*Ts  dataType=Inherit from 'Constant value'  isSigned=on  wordLen=16  udDataType=sfix(16)  fracBitsMode=Best precision  numFracBits=15  InterpretAs1D=-inf  Ts=-inf  FramebasedOutput=-inf
  Frame Conversion : FrameConversion  OutFrame=Sample-based
  Mean : dspstat3/Mean  run=off  reset_popup=None  InputProcessing=Columns as channels (frame based)  directionMode=Each column  dimension=1  treatSBRowAsCol=on  roiEnable=off  roiType=Rectangles  roiPortion=Entire ROI  roiOutput=Individual statistics for each ROI  roiFlag=off  outputDataTypeStr=Inherit: Same as accumulator  outputLastDataTypeStr=Inherit: Same as accumulator  outputMin=[]  outputMax=[]  roundingMode=Floor  overflowMode=off
  Product1 : Product  RndMeth=Zero
  Product2 : Product  Inputs=**  RndMeth=Zero
  Product3 : Product  Inputs=**  RndMeth=Zero
  Offset : Outport
  Slope : Outport  Port=2
  wires:
  Frame Conversion/1 -> Mean/1, Add2/2
  DSP Constant3/1 -> Product3/1
  DSP Constant2/1 -> Product1/2
  DSP Constant1/1 -> Product2/2
  Mean/1 -> Add2/1, Add4/1  "ybar"
  Add2/1 -> Product1/1  "yi-ybar"
  Product1/1 -> Add/1
  Add/1 -> Product2/1
  Product2/1 -> Product3/2, Slope/1  "b1"
  Product3/1 -> Add4/2  "b1*xbar"
  In1/1 -> Frame Conversion/1
  Add4/1 -> Offset/1  "b0"

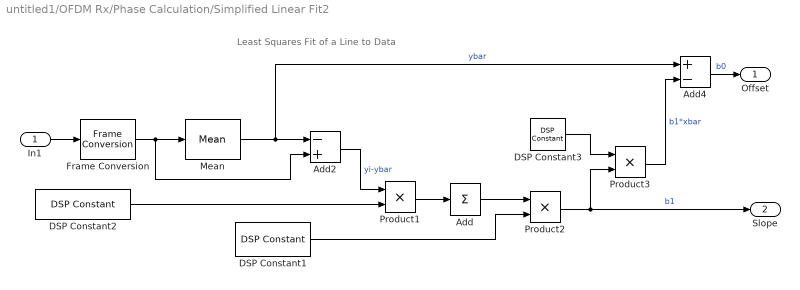
== system untitled1/OFDM Rx/Phase Calculation/Simplified Linear Fit2 ==
  note: Least Squares Fit of a Line to Data
  In1 : Inport
  Add : Sum  Inputs=+
  Add2 : Sum  Inputs=-+
  Add4 : Sum  Inputs=+-
  DSP Constant1 : dspobslib/DSP Constant  Value=1/14630  SampleMode=Discrete  discreteOutput=Sample-based  continuousOutput=Sample-based  sampTime=inf  framePeriod=N*Ts  dataType=Inherit from 'Constant value'  isSigned=on  wordLen=16  udDataType=sfix(16)  fracBitsMode=Best precision  numFracBits=15  InterpretAs1D=-inf  Ts=-inf  FramebasedOutput=-inf
  DSP Constant2 : dspobslib/DSP Constant  Value=[-27.5:27.5]'  SampleMode=Discrete  discreteOutput=Sample-based  continuousOutput=Sample-based  sampTime=inf  framePeriod=N*Ts  dataType=Inherit from 'Constant value'  isSigned=on  wordLen=16  udDataType=sfix(16)  fracBitsMode=Best precision  numFracBits=15  InterpretAs1D=-inf  Ts=-inf  FramebasedOutput=-inf
  DSP Constant3 : dspobslib/DSP Constant  Value=-.5  SampleMode=Discrete  discreteOutput=Sample-based  continuousOutput=Sample-based  sampTime=inf  framePeriod=N*Ts  dataType=Inherit from 'Constant value'  isSigned=on  wordLen=16  udDataType=sfix(16)  fracBitsMode=Best precision  numFracBits=15  InterpretAs1D=-inf  Ts=-inf  FramebasedOutput=-inf
  Frame Conversion : FrameConversion  OutFrame=Sample-based
  Mean : dspstat3/Mean  run=off  reset_popup=None  InputProcessing=Columns as channels (frame based)  directionMode=Each column  dimension=1  treatSBRowAsCol=on  roiEnable=off  roiType=Rectangles  roiPortion=Entire ROI  roiOutput=Individual statistics for each ROI  roiFlag=off  outputDataTypeStr=Inherit: Same as accumulator  outputLastDataTypeStr=Inherit: Same as accumulator  outputMin=[]  outputMax=[]  roundingMode=Floor  overflowMode=off
  Product1 : Product  RndMeth=Zero
  Product2 : Product  Inputs=**  RndMeth=Zero
  Product3 : Product  Inputs=**  RndMeth=Zero
  Offset : Outport
  Slope : Outport  Port=2
  wires:
  Add4/1 -> Offset/1  "b0"
  In1/1 -> Frame Conversion/1
  Product3/1 -> Add4/2  "b1*xbar"
  Product2/1 -> Slope/1, Product3/2  "b1"
  Add/1 -> Product2/1
  Product1/1 -> Add/1
  Add2/1 -> Product1/1  "yi-ybar"
  Mean/1 -> Add4/1, Add2/1  "ybar"
  DSP Constant1/1 -> Product2/2
  DSP Constant2/1 -> Product1/2
  DSP Constant3/1 -> Product3/1
  Frame Conversion/1 -> Add2/2, Mean/1

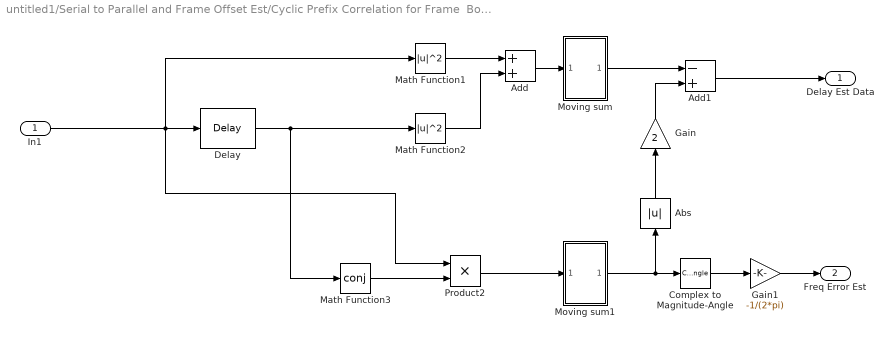
== system untitled1/Serial to Parallel and Frame Offset Est/Cyclic Prefix Correlation for Frame  Boundary Estimation/Estimators ==
  In1 : Inport
  Abs : Abs
  Add : Sum
  Add1 : Sum  Inputs=-+
  Complex to Magnitude-Angle : ComplexToMagnitudeAngle  Output=Angle
  Delay : dspsigops/Delay  InputProcessing=Inherited (this choice will be removed - see release notes)  dly_unit=Samples  delay=FFT_Size  ic_detail=off  dif_ic_for_ch=off  dif_ic_for_dly=off  ic=0  reset_popup=None
  Gain : Gain  Gain=2
  Gain1 : Gain  Gain=-1/(2*pi)
  Math Function1 : Math  Operator=magnitude^2  SaturateOnIntegerOverflow=on
  Math Function2 : Math  Operator=magnitude^2  SaturateOnIntegerOverflow=on
  Math Function3 : Math  Operator=conj  SaturateOnIntegerOverflow=on
  Moving sum : Subsystem
  Moving sum1 : Subsystem
  Product2 : Product  RndMeth=Zero
  Delay Est Data : Outport
  Freq Error Est : Outport  Port=2
  wires:
  In1/1 -> Product2/1, Delay/1, Math Function1/1
  Gain1/1 -> Freq Error Est/1
  Complex to Magnitude-Angle/1 -> Gain1/1
  Math Function3/1 -> Product2/2
  Gain/1 -> Add1/2
  Abs/1 -> Gain/1
  Add1/1 -> Delay Est Data/1
  Moving sum/1(Out1) -> Add1/1
  Moving sum1/1(Out1) -> Complex to Magnitude-Angle/1, Abs/1
  Product2/1 -> Moving sum1/1(In1)
  Add/1 -> Moving sum/1(In1)
  Math Function2/1 -> Add/2
  Math Function1/1 -> Add/1
  Delay/1 -> Math Function3/1, Math Function2/1

== system untitled1/Serial to Parallel and Frame Offset Est/Cyclic Prefix Correlation for Frame  Boundary Estimation/Find max ==
  In1 : Inport
  Enable : EnablePort
  Add : Sum  Inputs=+-
  Constant : Constant  Value=160/2
  Frame Conversion : FrameConversion  OutFrame=Sample-based
  Maximum : dspstat3/Maximum  fcn=Index  reset=None  InputProcessing=Columns as channels (frame based)  indexBase=One  operateOver=Each column  Dimension=1  colComp=on  operation=maximum  roiEnable=off  roiType=Rectangles  roiPortion=Entire ROI  roiOutput=Individual statistics for each ROI  roiFlag=off  accumDataTypeStr=Inherit: Same as product output  accumLastDataTypeStr=Inherit: Same as product output  roundingMode=Floor  overflowMode=off
  Moving sum : Subsystem
  reorder to center 0 point : Selector  InputPortWidth=160  IndexOptions=Index vector (dialog)  Indices=[(160/2+1):160 1:160/2]  OutputSizes=1
  Frame Offset Est : Outport  InitialOutput=0
  wires:
  In1/1 -> reorder to center 0 point/1
  Maximum/1 -> Frame Conversion/1
  reorder to center 0 point/1 -> Maximum/1
  Frame Conversion/1 -> Add/1
  Add/1 -> Moving sum/1(In1)
  Constant/1 -> Add/2
  Moving sum/1(Out1) -> Frame Offset Est/1

== system untitled1/Serial to Parallel and Frame Offset Est/Cyclic Prefix Correlation for Frame  Boundary Estimation/Estimators/Moving sum ==
  In1 : Inport
  Gain : Gain  Gain=1/Cyclic  SaturateOnIntegerOverflow=on  OutDataTypeStr=Inherit: Same as input  ParamDataTypeStr=Inherit: Same as input
  Integer Delay : Delay  DelayLength=Cyclic  InputProcessing=Inherited
  Integer Delay1 : Delay  DelayLength=1  InputProcessing=Inherited
  Sum2 : Sum  Inputs=|+-
  Sum3 : Sum  Inputs=|++
  Out1 : Outport
  wires:
  Gain/1 -> Out1/1
  In1/1 -> Sum2/1, Integer Delay/1
  Sum2/1 -> Sum3/1
  Integer Delay1/1 -> Sum3/2
  Sum3/1 -> Gain/1, Integer Delay1/1
  Integer Delay/1 -> Sum2/2

== system untitled1/Serial to Parallel and Frame Offset Est/Cyclic Prefix Correlation for Frame  Boundary Estimation/Estimators/Moving sum1 ==
  In1 : Inport
  Gain : Gain  Gain=1/Cyclic  SaturateOnIntegerOverflow=on  OutDataTypeStr=Inherit: Same as input  ParamDataTypeStr=Inherit: Same as input
  Integer Delay : Delay  DelayLength=Cyclic  InputProcessing=Inherited
  Integer Delay1 : Delay  DelayLength=1  InputProcessing=Inherited
  Sum2 : Sum  Inputs=|+-
  Sum3 : Sum  Inputs=|++
  Out1 : Outport
  wires:
  Integer Delay/1 -> Sum2/2
  Sum3/1 -> Integer Delay1/1, Gain/1
  Integer Delay1/1 -> Sum3/2
  Sum2/1 -> Sum3/1
  In1/1 -> Integer Delay/1, Sum2/1
  Gain/1 -> Out1/1

== system untitled1/Serial to Parallel and Frame Offset Est/Cyclic Prefix Correlation for Frame  Boundary Estimation/Find max/Moving sum ==
  In1 : Inport
  Gain : Gain  Gain=1/4  SaturateOnIntegerOverflow=on  OutDataTypeStr=Inherit: Same as input  ParamDataTypeStr=Inherit: Same as input
  Integer Delay : Delay  DelayLength=4  InputProcessing=Inherited
  Integer Delay1 : Delay  DelayLength=1  InitialCondition=0  InputProcessing=Inherited
  Sum2 : Sum  Inputs=|+-
  Sum3 : Sum  Inputs=|++
  Out1 : Outport
  wires:
  Integer Delay/1 -> Sum2/2
  Sum3/1 -> Integer Delay1/1, Gain/1
  Integer Delay1/1 -> Sum3/2
  Sum2/1 -> Sum3/1
  In1/1 -> Integer Delay/1, Sum2/1
  Gain/1 -> Out1/1
